simulink model "Cel2Fahr"  (R2016a)
settings: Solver=VariableStepAuto  StartTime=0.0  StopTime=10.0  RelTol=1e-3
settings Model: Creator=Islam Barakat  LastModifiedBy=Islam Barakat

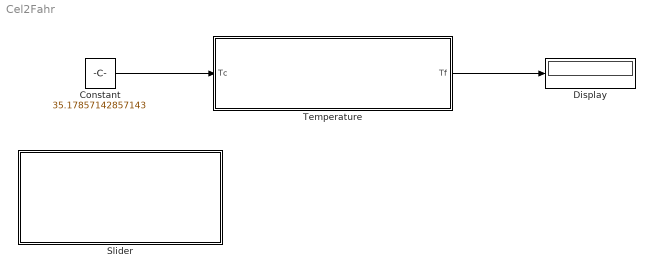
== system Cel2Fahr ==
  Constant : Constant  Value=35.17857142857143
  Display : Display
  Slider : Subsystem  DialogController=hmiCreateDDGDialog  IsWebBlock=on  mask(MWDashboardBlock){webBlockId=b7c66176-0e9a-4d82-93cc-e04dc23b4e48, webBlockType=slider, ShowInLibBrowser=on, ShowInitialText=on, HMISrcModelName=Cel2Fahr}
      mask prompts: webBlockId "WebBlock Id"; webBlockType "WebBlock Type"; HMISrcModelName "Source Model"
      mask Help: helpview([docroot '/mapfiles/simulink.map'], 'hmi_slider')
      mask Display:
      | if strcmp(get_param(bdroot(gcb),'BlockDiagramType'), 'library')
      |     image([(matlabroot) '/toolbox/simulink/hmi/icons/Slider.png']);
      | end
  Temperature : Subsystem
      mask Display:
      | set_param(gcbh,'BackgroundColor','Yellow');
      | 
      | disp('Temperature in Celisus to Fahrnheint');
  wires:
  Constant/1 -> Temperature/1(Tc)
  Temperature/1(Tf) -> Display/1

== system Cel2Fahr/Slider ==

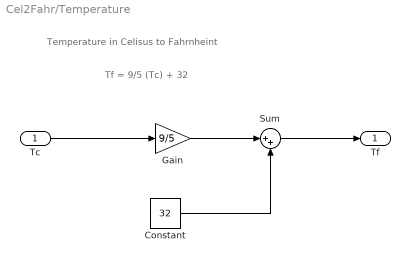
== system Cel2Fahr/Temperature ==
  note: Temperature in Celisus to Fahrnheint
  note: Tf = 9/5 (Tc) + 32
  Tc : Inport
  Constant : Constant  Value=32
      mask Display: set_param(gcbh,'BackgroundColor','Cyan');
  Gain : Gain  Gain=9/5
      mask Display: set_param(gcbh,'BackgroundColor','Cyan');
  Sum : Sum  Inputs=|++
  Tf : Outport
  wires:
  Tc/1 -> Gain/1
  Sum/1 -> Tf/1
  Gain/1 -> Sum/1
  Constant/1 -> Sum/2
